simulink model "sim_lqr"  (R2020a)
settings: Solver=VariableStepAuto  StartTime=0.0  StopTime=10.0  RelTol=1e-3
libraries: simulink x1
settings Model: Creator=10853  LastModifiedBy=yztk

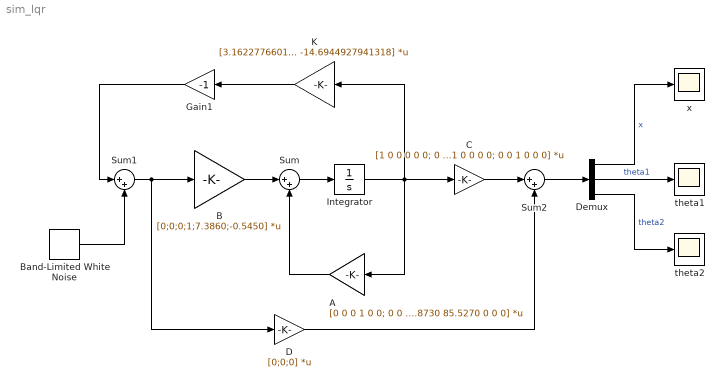
== system sim_lqr ==
  A : Gain  Gain=[0 0 0 1 0 0; 0 0 0 0 1 0; 0 0 0 0 0 1;0 0 0 0 0 0; 0 189.318 -116.9320 0 0 0; 0 -90.8730 85.5270 0 0 0]  Multiplication=Matrix(K*u)
  B : Gain  Gain=[0;0;0;1;7.3860;-0.5450]  Multiplication=Matrix(K*u)
  Band-Limited White Noise : simulink/Sources/Band-Limited White Noise  Cov=0.0005  Ts=0.01  seed=[23341]
  C : Gain  Gain=|  Multiplication=Matrix(K*u)
      | [1 0 0 0 0 0;
      | 0 1 0 0 0 0;
      | 0 0 1 0 0 0]
  D : Gain  Gain=[0;0;0]  Multiplication=Matrix(K*u)
  Demux : Demux  Outputs=3
  Gain1 : Gain  Gain=-1
  Integrator : Integrator  InitialCondition=[0 5*pi/180 5*pi/180 0 0 0]
  K : Gain  Gain="[3.16227766016844\t119.515654610910\t-138.616735557833\t4.31948065674680\t4.26792956895651\t-14.6944927941318]"  Multiplication=Matrix(K*u)
  Sum : Sum  Inputs=|++
  Sum1 : Sum  Inputs=|++
  Sum2 : Sum  Inputs=|++
  theta1 : Scope
  theta2 : Scope
  x : Scope
  wires:
  B/1 -> Sum/1
  Sum/1 -> Integrator/1
  A/1 -> Sum/2
  Integrator/1 -> A/1, C/1, K/1
  Demux/1 -> x/1  "x"
  Demux/2 -> theta1/1  "theta1"
  Demux/3 -> theta2/1  "theta2"
  K/1 -> Gain1/1
  Gain1/1 -> Sum1/1
  Band-Limited White Noise/1 -> Sum1/2
  D/1 -> Sum2/2
  Sum1/1 -> D/1, B/1
  Sum2/1 -> Demux/1
  C/1 -> Sum2/1
